simulink model "LKA_ensemble_RL_training"  (R2022a)
settings: Solver=FixedStepAuto  StartTime=0.0  StopTime=T  FixedStep=Ts  RelTol=1e-3
undefined symbols (not defined in the file): actionTable, actionUB, Cf, Cr, DiscIntNeverNeededParam, e1_initial, e2_initial, isEnsembleTerminate, isPred, isTerminate, Iz, lat_terminate_error, lf, lr, m, max_late_dev, max_rel_yaw_ang, md, rewardToIndex, rewardUB1, rewardUB2, rewardWeights, stateTable, tranTable, Ts, u_max, u_min, Vx
libraries: rllib x10, simulink x2
settings Model: Creator=The MathWorks, Inc.  LastModifiedBy=jiayangsong
settings SolverCC: AlgebraicLoopSolver=TrustRegion
settings DataIOCC: ReturnWorkspaceOutputs=off
settings DebuggingCC: UnconnectedInputMsg=warning  UnconnectedOutputMsg=warning  UnconnectedLineMsg=warning  SFMachineParentedDataDiag=warning  ArithmeticOperatorsInVariantConditions=warning
settings SFSimCC: SimUseLocalCustomCode=off  CustomCodeUndefinedFunction=UseInterfaceOnly
settings RTWCC: RTWUseLocalCustomCode=off  DLArmComputeVersion=19.05
settings CodeAppCC: StateflowObjectComments=on
settings SimscapeCC: SimscapeNormalizeSystem=off

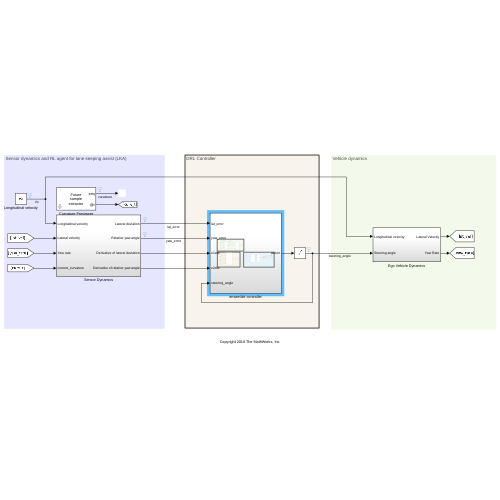
[thumbnail: Simulink's stored preview of the top-level diagram]
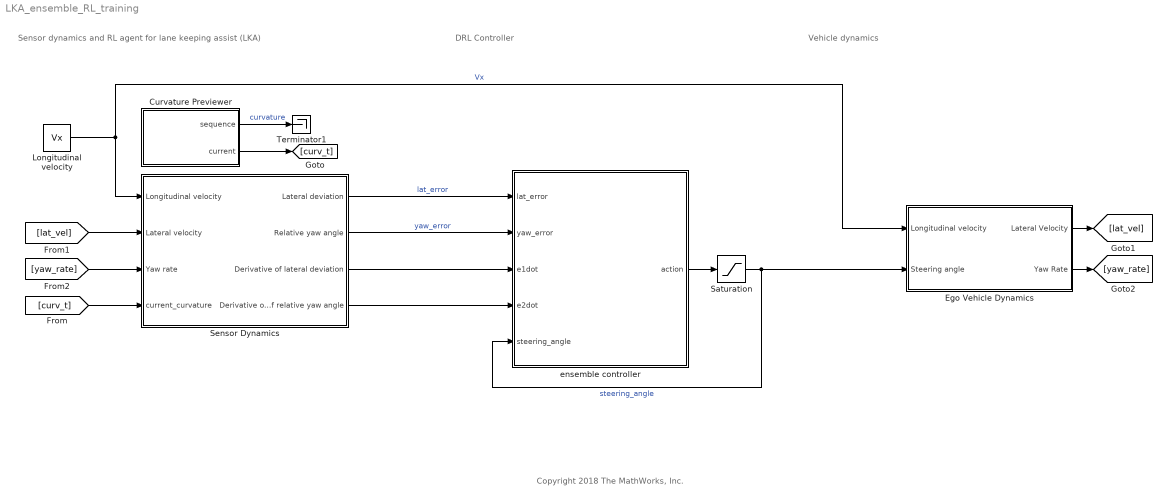
== system LKA_ensemble_RL_training ==
  note: DRL Controller
  note: Vehicle dynamics
  note: Sensor dynamics and RL agent for lane keeping assist (LKA)
  note: Copyright 2018 The MathWorks, Inc.
  Curvature Previewer : Subsystem  mask{signal=md, ts=Ts, steps=10}
      mask prompts: signal "Signal name"; ts "Sampling time"; steps "Number of previewing steps"
      mask init:
      | ts = evalin('base',get_param(gcbh,'ts'));
      | signal = evalin('base',get_param(gcbh,'signal'));
      | steps = evalin('base',get_param(gcbh,'steps'));
      | data = mpc_previewer_maskinit(signal,ts);
      mask Display:
      | fprintf('Future\nsample\nextractor');
      | port_label('output', 1, 'seq')
      | port_label('output', 2, '@t')
  Ego Vehicle Dynamics : Subsystem
  Longitudinal velocity : Constant  Value=Vx  SampleTime=Ts
  Saturation : Saturate  UpperLimit=u_max  LowerLimit=u_min
  Sensor Dynamics : Subsystem
  Terminator1 : Terminator
  ensemble controller : Subsystem
  wires:
  Ego Vehicle Dynamics/1(Lateral Velocity) -> [lat_vel]
  Longitudinal velocity/1 -> Ego Vehicle Dynamics/1(Longitudinal velocity), Sensor Dynamics/1(Longitudinal velocity)  "Vx"
  Curvature Previewer/2(current) -> [curv_t]
  [curv_t] -> Sensor Dynamics/4(current_curvature)
  Ego Vehicle Dynamics/2(Yaw Rate) -> [yaw_rate]
  [lat_vel] -> Sensor Dynamics/2(Lateral velocity)
  [yaw_rate] -> Sensor Dynamics/3(Yaw rate)
  Saturation/1 -> Ego Vehicle Dynamics/2(Steering angle), ensemble controller/5(steering_angle)  "steering_angle"
  Curvature Previewer/1(sequence) -> Terminator1/1  "curvature"
  Sensor Dynamics/1(Lateral deviation) -> ensemble controller/1(lat_error)  "lat_error"
  Sensor Dynamics/2(Relative yaw angle) -> ensemble controller/2(yaw_error)  "yaw_error"
  Sensor Dynamics/3(Derivative of lateral deviation) -> ensemble controller/3("e1dot ")
  Sensor Dynamics/4(Derivative of relative yaw angle) -> ensemble controller/4(e2dot)
  ensemble controller/1(action) -> Saturation/1

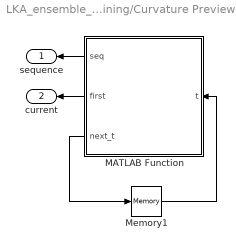
== system LKA_ensemble_RL_training/Curvature Previewer ==
  MATLAB Function : MATLAB Function  TreatAsAtomicUnit=on
  Memory1 : Memory  InheritSampleTime=on  LinearizeAsDelay=on
  sequence : Outport  VectorParamsAs1DForOutWhenUnconnected=off
  current : Outport  Port=2  VectorParamsAs1DForOutWhenUnconnected=off
  wires:
  MATLAB Function/1(seq) -> sequence/1
  MATLAB Function/2(first) -> current/1
  Memory1/1 -> MATLAB Function/1(t)
  MATLAB Function/3(next_t) -> Memory1/1

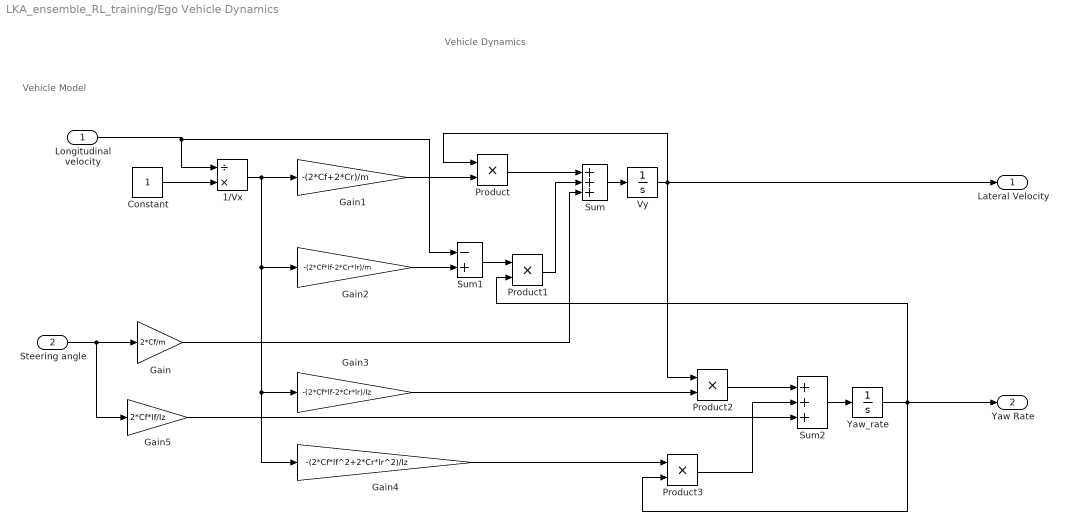
== system LKA_ensemble_RL_training/Ego Vehicle Dynamics ==
  note: Vehicle Model
  note: Vehicle Dynamics
  Longitudinal velocity : Inport
  Steering angle : Inport  Port=2
  1/Vx : Product  Inputs=/*
  Constant : Constant
  Gain : Gain  Gain=2*Cf/m
  Gain1 : Gain  Gain=-(2*Cf+2*Cr)/m
  Gain2 : Gain  Gain=-(2*Cf*lf-2*Cr*lr)/m
  Gain3 : Gain  Gain=-(2*Cf*lf-2*Cr*lr)/Iz
  Gain4 : Gain  Gain=-(2*Cf*lf^2+2*Cr*lr^2)/Iz
  Gain5 : Gain  Gain=2*Cf*lf/Iz
  Product{,1..3} (4 alike) : Product
  Sum : Sum  Inputs=+++
  Sum1 : Sum  Inputs=-+
  Sum2 : Sum  Inputs=+++
  Vy : Integrator
  "Yaw_rate " : Integrator
  Lateral Velocity : Outport  VectorParamsAs1DForOutWhenUnconnected=off
  Yaw Rate : Outport  Port=2  VectorParamsAs1DForOutWhenUnconnected=off
  wires:
  Sum2/1 -> "Yaw_rate "/1
  Gain2/1 -> Sum1/2
  Gain4/1 -> Product3/1
  Constant/1 -> 1/Vx/2
  Gain3/1 -> Product2/2
  1/Vx/1 -> Gain4/1, Gain3/1, Gain2/1, Gain1/1
  Product2/1 -> Sum2/1
  Product3/1 -> Sum2/2
  Gain5/1 -> Sum2/3
  Sum1/1 -> Product1/1
  "Yaw_rate "/1 -> Product3/2, Yaw Rate/1, Product1/2
  Gain/1 -> Sum/3
  Steering angle/1 -> Gain/1, Gain5/1
  Gain1/1 -> Product/2
  Product/1 -> Sum/1
  Vy/1 -> Product/1, Lateral Velocity/1, Product2/1
  Sum/1 -> Vy/1
  Longitudinal velocity/1 -> Sum1/1, 1/Vx/1
  Product1/1 -> Sum/2

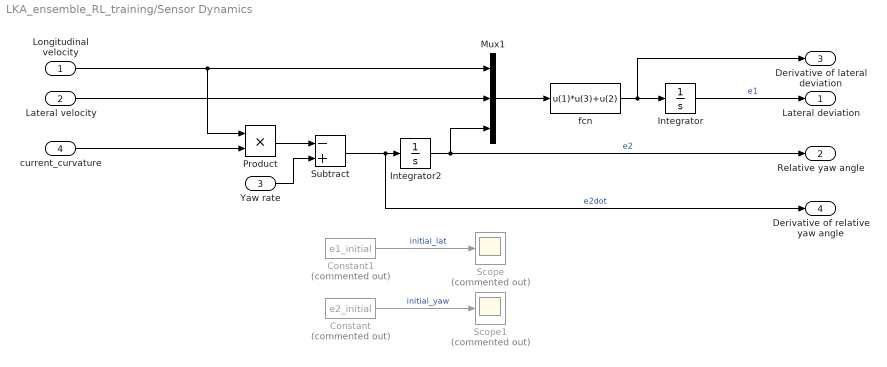
== system LKA_ensemble_RL_training/Sensor Dynamics ==
  Longitudinal velocity : Inport
  Lateral velocity : Inport  Port=2
  Yaw rate : Inport  Port=3
  current_curvature : Inport  Port=4
  Constant : Constant  Commented=on  Value=e2_initial
  Constant1 : Constant  Commented=on  Value=e1_initial
  Integrator : Integrator  InitialCondition=e1_initial
  Integrator2 : Integrator  InitialCondition=e2_initial
  Mux1 : Mux  Inputs=[1 1 1]
  Product : Product
  Scope : Scope  Commented=on
  Scope1 : Scope  Commented=on
  Subtract : Sum  Inputs=-+
  fcn : Fcn  Expr=u(1)*u(3)+u(2)
  Lateral deviation : Outport  VectorParamsAs1DForOutWhenUnconnected=off
  Relative yaw angle : Outport  Port=2  VectorParamsAs1DForOutWhenUnconnected=off
  Derivative of lateral deviation : Outport  Port=3  VectorParamsAs1DForOutWhenUnconnected=off
  Derivative of relative yaw angle : Outport  Port=4  VectorParamsAs1DForOutWhenUnconnected=off
  wires:
  Integrator2/1 -> Relative yaw angle/1, Mux1/3  "e2"
  Mux1/1 -> fcn/1
  fcn/1 -> Derivative of lateral deviation/1, Integrator/1
  Lateral velocity/1 -> Mux1/2
  Integrator/1 -> Lateral deviation/1  "e1"
  Product/1 -> Subtract/1
  Yaw rate/1 -> Subtract/2
  Subtract/1 -> Derivative of relative yaw angle/1, Integrator2/1  "e2dot"
  Longitudinal velocity/1 -> Mux1/1, Product/1
  current_curvature/1 -> Product/2
  Constant1/1 -> Scope/1  "initial_lat"
  Constant/1 -> Scope1/1  "initial_yaw"

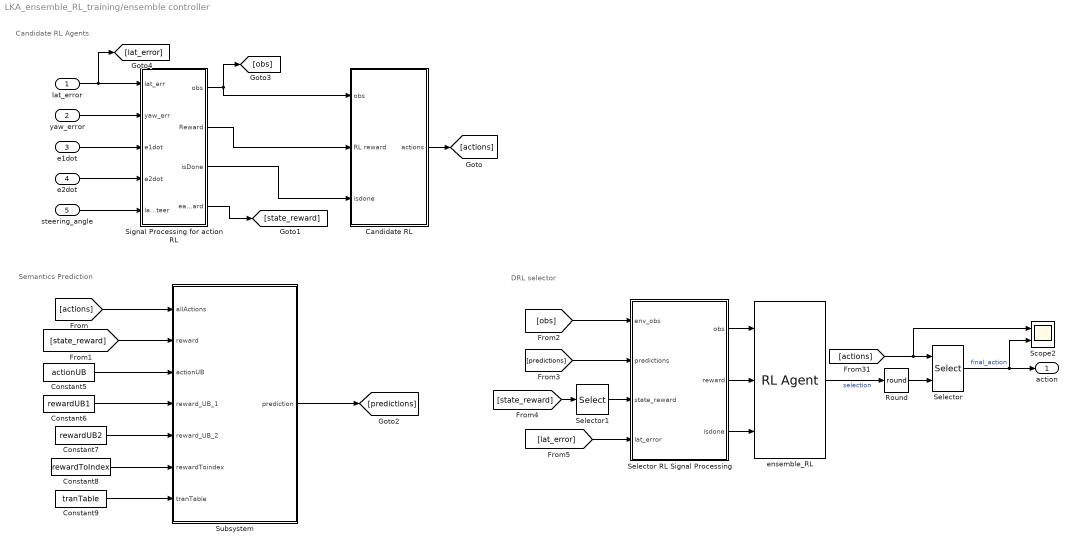
== system LKA_ensemble_RL_training/ensemble controller ==
  note: DRL selector
  note: Semantics Prediction
  note: Candidate RL Agents
  lat_error : Inport
  yaw_error : Inport  Port=2
  "e1dot " : Inport  Port=3
  e2dot : Inport  Port=4
  steering_angle : Inport  Port=5
  Candidate RL : Subsystem
  Constant5 : Constant  Value=actionUB
  Constant6 : Constant  Value=rewardUB1
  Constant7 : Constant  Value=rewardUB2
  Constant8 : Constant  Value=rewardToIndex
  Constant9 : Constant  Value=tranTable
  Round : Rounding  Operator=round
  Scope2 : Scope  NumInputPorts=2
  Selector : Selector  IndexOptions=Index vector (port)  Indices=[1 3]  OutputSizes=1
  Selector RL Signal Processing : Subsystem
  Selector1 : Selector  InputPortWidth=3  IndexOptions=Index vector (dialog)  Indices=[3]  OutputSizes=1
  "Signal Processing for action RL " : Subsystem
  Subsystem : Subsystem
  ensemble_RL : rllib/RL Agent  Agent=agentEnsemble  ExternalActionAsInput=off  ProvideLastAction=off  ProvideCumRwd=off  TreatAsDirectFeedthrough=on  UseStrictObservationDataTypes=off
  action : Outport
  wires:
  yaw_error/1 -> "Signal Processing for action RL "/2(yaw_err)
  e2dot/1 -> "Signal Processing for action RL "/4(e2dot)
  steering_angle/1 -> "Signal Processing for action RL "/5(last_RL_steer)
  "e1dot "/1 -> "Signal Processing for action RL "/3("e1dot ")
  lat_error/1 -> [lat_error], "Signal Processing for action RL "/1(lat_err)
  "Signal Processing for action RL "/1(obs) -> Candidate RL/1(obs), [obs]
  "Signal Processing for action RL "/2(Reward) -> Candidate RL/2(RL reward)
  "Signal Processing for action RL "/3(isDone) -> Candidate RL/3(isdone)
  Candidate RL/1(actions) -> [actions]
  [actions] -> Subsystem/1(allActions)
  [state_reward] -> Subsystem/2(reward)
  Constant5/1 -> Subsystem/3(actionUB)
  Constant7/1 -> Subsystem/5(reward_UB_2)
  Constant6/1 -> Subsystem/4(reward_UB_1)
  Constant8/1 -> Subsystem/6(rewardToindex)
  Constant9/1 -> Subsystem/7(tranTable)
  ensemble_RL/1 -> Round/1  "selection"
  Round/1 -> Selector/2
  [actions] -> Scope2/1, Selector/1
  Selector/1 -> Scope2/2, action/1  "final_action"
  Selector RL Signal Processing/1(obs) -> ensemble_RL/1
  Selector RL Signal Processing/2(reward) -> ensemble_RL/2
  Selector RL Signal Processing/3(isdone) -> ensemble_RL/3
  [obs] -> Selector RL Signal Processing/1(env_obs)
  [predictions] -> Selector RL Signal Processing/2(predictions)
  [lat_error] -> Selector RL Signal Processing/4(lat_error)
  Subsystem/1(prediction) -> [predictions]
  "Signal Processing for action RL "/4(each_reward) -> [state_reward]
  [state_reward] -> Selector1/1
  Selector1/1 -> Selector RL Signal Processing/3(state_reward)

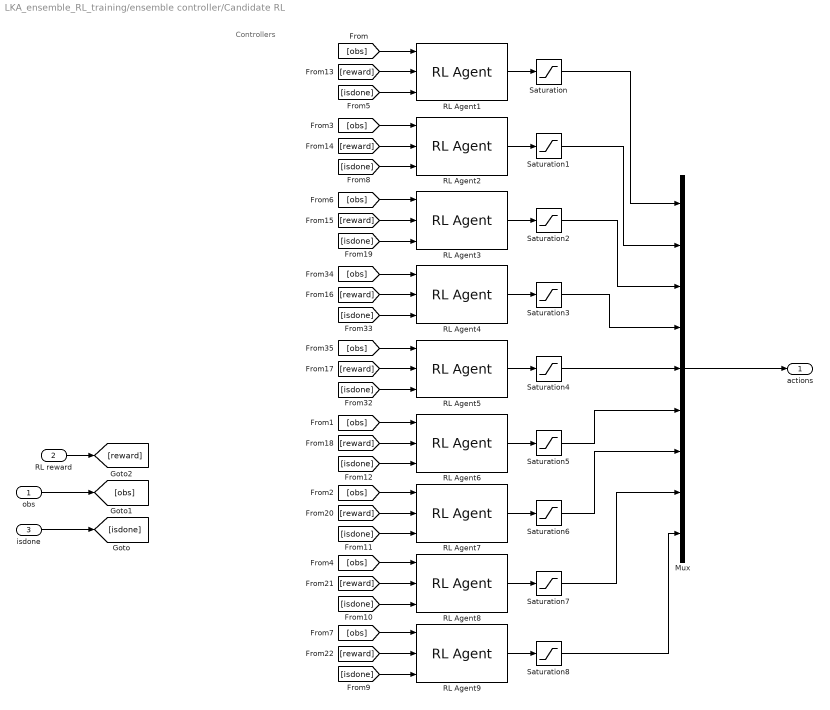
== system LKA_ensemble_RL_training/ensemble controller/Candidate RL ==
  note: Controllers
  obs : Inport
  RL reward : Inport  Port=2
  isdone : Inport  Port=3
  Mux : Mux  Inputs=9
  RL Agent1 : rllib/RL Agent  Agent=agent1  ExternalActionAsInput=off  ProvideLastAction=off  ProvideCumRwd=off  TreatAsDirectFeedthrough=on  UseStrictObservationDataTypes=off
  RL Agent2 : rllib/RL Agent  Agent=agent2  ExternalActionAsInput=off  ProvideLastAction=off  ProvideCumRwd=off  TreatAsDirectFeedthrough=on  UseStrictObservationDataTypes=off
  RL Agent3 : rllib/RL Agent  Agent=agent3  ExternalActionAsInput=off  ProvideLastAction=off  ProvideCumRwd=off  TreatAsDirectFeedthrough=on  UseStrictObservationDataTypes=off
  RL Agent4 : rllib/RL Agent  Agent=agent3  ExternalActionAsInput=off  ProvideLastAction=off  ProvideCumRwd=off  TreatAsDirectFeedthrough=on  UseStrictObservationDataTypes=off
  RL Agent5 : rllib/RL Agent  Agent=agent3  ExternalActionAsInput=off  ProvideLastAction=off  ProvideCumRwd=off  TreatAsDirectFeedthrough=on  UseStrictObservationDataTypes=off
  RL Agent6 : rllib/RL Agent  Agent=agent6  ExternalActionAsInput=off  ProvideLastAction=off  ProvideCumRwd=off  TreatAsDirectFeedthrough=on  UseStrictObservationDataTypes=off
  RL Agent7 : rllib/RL Agent  Agent=agent7  ExternalActionAsInput=off  ProvideLastAction=off  ProvideCumRwd=off  TreatAsDirectFeedthrough=on  UseStrictObservationDataTypes=off
  RL Agent8 : rllib/RL Agent  Agent=agent8  ExternalActionAsInput=off  ProvideLastAction=off  ProvideCumRwd=off  TreatAsDirectFeedthrough=on  UseStrictObservationDataTypes=off
  RL Agent9 : rllib/RL Agent  Agent=agent9  ExternalActionAsInput=off  ProvideLastAction=off  ProvideCumRwd=off  TreatAsDirectFeedthrough=on  UseStrictObservationDataTypes=off
  Saturation{,1..8} (9 alike) : Saturate  UpperLimit=u_max  LowerLimit=u_min
  actions : Outport
  wires:
  [obs] -> RL Agent7/1
  [obs] -> RL Agent4/1
  [obs] -> RL Agent3/1
  Saturation3/1 -> Mux/4
  [obs] -> RL Agent1/1
  [isdone] -> RL Agent1/3
  [obs] -> RL Agent2/1
  [obs] -> RL Agent5/1
  RL Agent1/1 -> Saturation/1
  [isdone] -> RL Agent8/3
  [isdone] -> RL Agent6/3
  Saturation/1 -> Mux/1
  RL Agent6/1 -> Saturation5/1
  Saturation4/1 -> Mux/5
  RL Agent3/1 -> Saturation2/1
  [isdone] -> RL Agent2/3
  [isdone] -> RL Agent7/3
  RL Agent8/1 -> Saturation7/1
  Saturation1/1 -> Mux/2
  [isdone] -> RL Agent5/3
  Mux/1 -> actions/1
  [obs] -> RL Agent6/1
  [isdone] -> RL Agent3/3
  RL Agent5/1 -> Saturation4/1
  RL Agent4/1 -> Saturation3/1
  RL Agent7/1 -> Saturation6/1
  RL Agent2/1 -> Saturation1/1
  [obs] -> RL Agent8/1
  Saturation2/1 -> Mux/3
  [isdone] -> RL Agent4/3
  RL Agent9/1 -> Saturation8/1
  [obs] -> RL Agent9/1
  [isdone] -> RL Agent9/3
  Saturation5/1 -> Mux/6
  Saturation6/1 -> Mux/7
  Saturation7/1 -> Mux/8
  Saturation8/1 -> Mux/9
  isdone/1 -> [isdone]
  obs/1 -> [obs]
  RL reward/1 -> [reward]
  [reward] -> RL Agent1/2
  [reward] -> RL Agent2/2
  [reward] -> RL Agent3/2
  [reward] -> RL Agent4/2
  [reward] -> RL Agent5/2
  [reward] -> RL Agent6/2
  [reward] -> RL Agent7/2
  [reward] -> RL Agent8/2
  [reward] -> RL Agent9/2

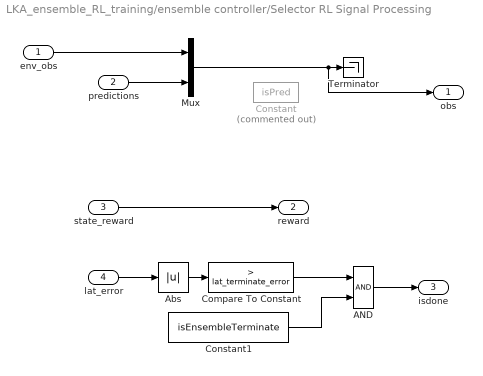
== system LKA_ensemble_RL_training/ensemble controller/Selector RL Signal Processing ==
  env_obs : Inport
  predictions : Inport  Port=2
  state_reward : Inport  Port=3
  lat_error : Inport  Port=4
  AND : Logic  IconShape=distinctive  AllPortsSameDT=off  OutDataTypeStr=boolean
  Abs : Abs  SaturateOnIntegerOverflow=off
  Compare To Constant : simulink/Logic and Bit Operations/Compare To Constant  relop=>  const=lat_terminate_error  OutDataTypeStr=boolean
  Constant : Constant  Commented=on  Value=isPred
  Constant1 : Constant  Value=isEnsembleTerminate
  Mux : Mux  Inputs=2
  Terminator : Terminator
  obs : Outport
  reward : Outport  Port=2
  isdone : Outport  Port=3
  wires:
  state_reward/1 -> reward/1
  Compare To Constant/1 -> AND/1
  Constant1/1 -> AND/2
  AND/1 -> isdone/1
  Abs/1 -> Compare To Constant/1
  lat_error/1 -> Abs/1
  predictions/1 -> Mux/2
  env_obs/1 -> Mux/1
  Mux/1 -> obs/1, Terminator/1

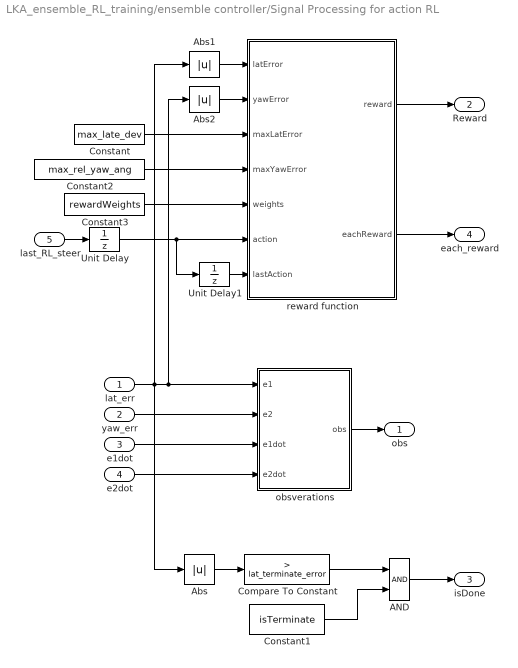
== system LKA_ensemble_RL_training/ensemble controller/Signal Processing for action RL  ==
  lat_err : Inport
  yaw_err : Inport  Port=2
  "e1dot " : Inport  Port=3
  e2dot : Inport  Port=4
  last_RL_steer : Inport  Port=5
  AND : Logic  IconShape=distinctive  AllPortsSameDT=off  OutDataTypeStr=boolean
  Abs : Abs  SaturateOnIntegerOverflow=off
  Abs1 : Abs  SaturateOnIntegerOverflow=off
  Abs2 : Abs  SaturateOnIntegerOverflow=off
  Compare To Constant : simulink/Logic and Bit Operations/Compare To Constant  relop=>  const=lat_terminate_error  OutDataTypeStr=boolean
  Constant : Constant  Value=max_late_dev
  Constant1 : Constant  Value=isTerminate
  Constant2 : Constant  Value=max_rel_yaw_ang
  Constant3 : Constant  Value=rewardWeights
  Unit Delay : UnitDelay  SampleTime=-1  HasFrameUpgradeWarning=on
  Unit Delay1 : UnitDelay  SampleTime=-1  HasFrameUpgradeWarning=on
  obsverations : Subsystem
  reward function : MATLAB Function  TreatAsAtomicUnit=on
  obs : Outport  VectorParamsAs1DForOutWhenUnconnected=off
  Reward : Outport  Port=2  VectorParamsAs1DForOutWhenUnconnected=off
  isDone : Outport  Port=3  VectorParamsAs1DForOutWhenUnconnected=off
  each_reward : Outport  Port=4
  wires:
  obsverations/1(obs) -> obs/1
  "e1dot "/1 -> obsverations/3(e1dot)
  e2dot/1 -> obsverations/4(e2dot)
  yaw_err/1 -> obsverations/2(e2)
  lat_err/1 -> obsverations/1(e1), Abs2/1, Abs1/1, Abs/1
  reward function/1(reward) -> Reward/1
  Constant/1 -> reward function/3(maxLatError)
  Abs1/1 -> reward function/1(latError)
  Abs2/1 -> reward function/2(yawError)
  last_RL_steer/1 -> Unit Delay/1
  Abs/1 -> Compare To Constant/1
  Compare To Constant/1 -> AND/1
  Constant1/1 -> AND/2
  AND/1 -> isDone/1
  Constant3/1 -> reward function/5(weights)
  Unit Delay1/1 -> reward function/7(lastAction)
  Constant2/1 -> reward function/4(maxYawError)
  Unit Delay/1 -> Unit Delay1/1, reward function/6(action)
  reward function/2(eachReward) -> each_reward/1

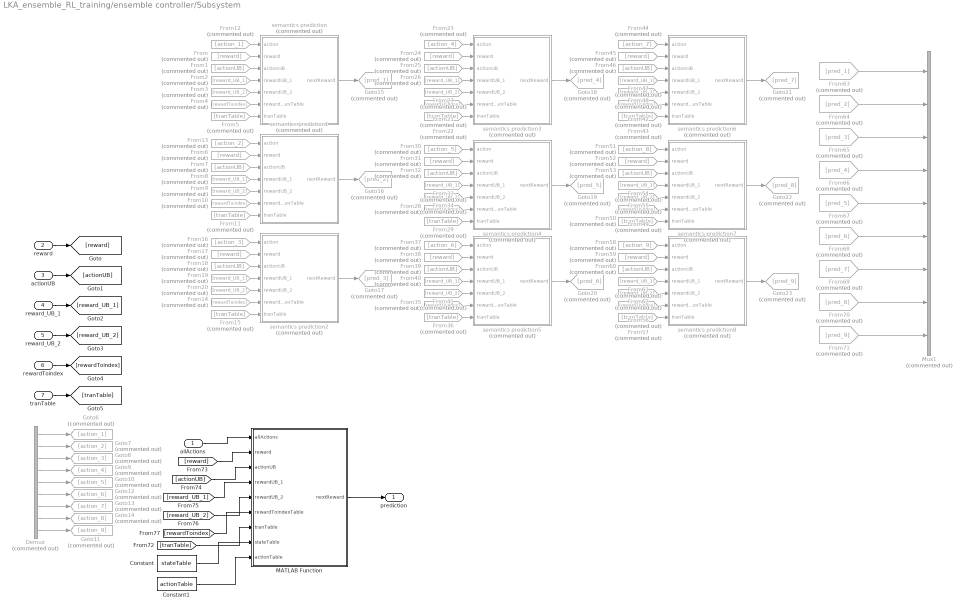
== system LKA_ensemble_RL_training/ensemble controller/Subsystem ==
  allActions : Inport
  reward : Inport  Port=2
  actionUB : Inport  Port=3
  reward_UB_1 : Inport  Port=4
  reward_UB_2 : Inport  Port=5
  rewardToindex : Inport  Port=6
  tranTable : Inport  Port=7
  Constant : Constant  Value=stateTable
  Constant1 : Constant  Value=actionTable
  Demux : Demux  Commented=on  Outputs=9
  From{,6,17,24,31,38,45,52,59} (9 alike) : From  Commented=on  GotoTag=reward
  From{1,7,18,25,32,39,46,53,60} (9 alike) : From  Commented=on  GotoTag=actionUB
  From{4,10,14,21,28,35,42,49,56} (9 alike) : From  Commented=on  GotoTag=rewardToindex
  From{5,11,15,22,29,36,43,50,57} (9 alike) : From  Commented=on  GotoTag=tranTable
  From12 : From  Commented=on  GotoTag=action_1
  From13 : From  Commented=on  GotoTag=action_2
  From16 : From  Commented=on  GotoTag=action_3
  From{2,8,19,26,33,40,47,54,61} (9 alike) : From  Commented=on  GotoTag=reward_UB_1
  From{3,9,20,27,34,41,48,55,62} (9 alike) : From  Commented=on  GotoTag=reward_UB_2
  From23 : From  Commented=on  GotoTag=action_4
  From30 : From  Commented=on  GotoTag=action_5
  From37 : From  Commented=on  GotoTag=action_6
  From44 : From  Commented=on  GotoTag=action_7
  From51 : From  Commented=on  GotoTag=action_8
  From58 : From  Commented=on  GotoTag=action_9
  From63 : From  Commented=on  GotoTag=pred_1
  From64 : From  Commented=on  GotoTag=pred_2
  From65 : From  Commented=on  GotoTag=pred_3
  From66 : From  Commented=on  GotoTag=pred_4
  From67 : From  Commented=on  GotoTag=pred_5
  From68 : From  Commented=on  GotoTag=pred_6
  From69 : From  Commented=on  GotoTag=pred_7
  From70 : From  Commented=on  GotoTag=pred_8
  From71 : From  Commented=on  GotoTag=pred_9
  Goto10 : Goto  Commented=on  GotoTag=action_5
  Goto11 : Goto  Commented=on  GotoTag=action_9
  Goto12 : Goto  Commented=on  GotoTag=action_6
  Goto13 : Goto  Commented=on  GotoTag=action_7
  Goto14 : Goto  Commented=on  GotoTag=action_8
  Goto15 : Goto  Commented=on  GotoTag=pred_1
  Goto16 : Goto  Commented=on  GotoTag=pred_2
  Goto17 : Goto  Commented=on  GotoTag=pred_3
  Goto18 : Goto  Commented=on  GotoTag=pred_4
  Goto19 : Goto  Commented=on  GotoTag=pred_5
  Goto20 : Goto  Commented=on  GotoTag=pred_6
  Goto21 : Goto  Commented=on  GotoTag=pred_7
  Goto22 : Goto  Commented=on  GotoTag=pred_8
  Goto23 : Goto  Commented=on  GotoTag=pred_9
  Goto6 : Goto  Commented=on  GotoTag=action_1
  Goto7 : Goto  Commented=on  GotoTag=action_2
  Goto8 : Goto  Commented=on  GotoTag=action_3
  Goto9 : Goto  Commented=on  GotoTag=action_4
  MATLAB Function : MATLAB Function  TreatAsAtomicUnit=on
  Mux1 : Mux  Commented=on  Inputs=9
  semantics prediction : MATLAB Function  Commented=on  TreatAsAtomicUnit=on
  semantics prediction1 : MATLAB Function  Commented=on  TreatAsAtomicUnit=on
  semantics prediction2 : MATLAB Function  Commented=on  TreatAsAtomicUnit=on
  semantics prediction3 : MATLAB Function  Commented=on  TreatAsAtomicUnit=on
  semantics prediction4 : MATLAB Function  Commented=on  TreatAsAtomicUnit=on
  semantics prediction5 : MATLAB Function  Commented=on  TreatAsAtomicUnit=on
  semantics prediction6 : MATLAB Function  Commented=on  TreatAsAtomicUnit=on
  semantics prediction7 : MATLAB Function  Commented=on  TreatAsAtomicUnit=on
  semantics prediction8 : MATLAB Function  Commented=on  TreatAsAtomicUnit=on
  prediction : Outport
  wires:
  reward/1 -> [reward]
  From/1 -> semantics prediction/2(reward)
  From63/1 -> Mux1/1
  From64/1 -> Mux1/2
  From65/1 -> Mux1/3
  From66/1 -> Mux1/4
  From67/1 -> Mux1/5
  From68/1 -> Mux1/6
  From69/1 -> Mux1/7
  From70/1 -> Mux1/8
  From71/1 -> Mux1/9
  actionUB/1 -> [actionUB]
  reward_UB_1/1 -> [reward_UB_1]
  reward_UB_2/1 -> [reward_UB_2]
  rewardToindex/1 -> [rewardToindex]
  tranTable/1 -> [tranTable]
  From1/1 -> semantics prediction/3(actionUB)
  From2/1 -> semantics prediction/4(rewardUB_1)
  From3/1 -> semantics prediction/5(rewardUB_2)
  From4/1 -> semantics prediction/6(rewardToIndexTable)
  From5/1 -> semantics prediction/7(tranTable)
  From9/1 -> semantics prediction1/5(rewardUB_2)
  From11/1 -> semantics prediction1/7(tranTable)
  From6/1 -> semantics prediction1/2(reward)
  From7/1 -> semantics prediction1/3(actionUB)
  From10/1 -> semantics prediction1/6(rewardToIndexTable)
  From8/1 -> semantics prediction1/4(rewardUB_1)
  Demux/1 -> Goto6/1
  Demux/2 -> Goto7/1
  Demux/3 -> Goto8/1
  Demux/4 -> Goto9/1
  Demux/5 -> Goto10/1
  Demux/6 -> Goto12/1
  Demux/7 -> Goto13/1
  Demux/8 -> Goto14/1
  Demux/9 -> Goto11/1
  From12/1 -> semantics prediction/1(action)
  From13/1 -> semantics prediction1/1(action)
  From16/1 -> semantics prediction2/1(action)
  From18/1 -> semantics prediction2/3(actionUB)
  From19/1 -> semantics prediction2/4(rewardUB_1)
  From14/1 -> semantics prediction2/6(rewardToIndexTable)
  From15/1 -> semantics prediction2/7(tranTable)
  From17/1 -> semantics prediction2/2(reward)
  From20/1 -> semantics prediction2/5(rewardUB_2)
  From23/1 -> semantics prediction3/1(action)
  From25/1 -> semantics prediction3/3(actionUB)
  From26/1 -> semantics prediction3/4(rewardUB_1)
  From21/1 -> semantics prediction3/6(rewardToIndexTable)
  From22/1 -> semantics prediction3/7(tranTable)
  From24/1 -> semantics prediction3/2(reward)
  From27/1 -> semantics prediction3/5(rewardUB_2)
  From30/1 -> semantics prediction4/1(action)
  From32/1 -> semantics prediction4/3(actionUB)
  From33/1 -> semantics prediction4/4(rewardUB_1)
  From28/1 -> semantics prediction4/6(rewardToIndexTable)
  From29/1 -> semantics prediction4/7(tranTable)
  From31/1 -> semantics prediction4/2(reward)
  From34/1 -> semantics prediction4/5(rewardUB_2)
  From37/1 -> semantics prediction5/1(action)
  From39/1 -> semantics prediction5/3(actionUB)
  From40/1 -> semantics prediction5/4(rewardUB_1)
  From35/1 -> semantics prediction5/6(rewardToIndexTable)
  From36/1 -> semantics prediction5/7(tranTable)
  From38/1 -> semantics prediction5/2(reward)
  From41/1 -> semantics prediction5/5(rewardUB_2)
  From50/1 -> semantics prediction7/7(tranTable)
  From53/1 -> semantics prediction7/3(actionUB)
  From52/1 -> semantics prediction7/2(reward)
  From47/1 -> semantics prediction6/4(rewardUB_1)
  From62/1 -> semantics prediction8/5(rewardUB_2)
  From56/1 -> semantics prediction8/6(rewardToIndexTable)
  From59/1 -> semantics prediction8/2(reward)
  From46/1 -> semantics prediction6/3(actionUB)
  From42/1 -> semantics prediction6/6(rewardToIndexTable)
  From57/1 -> semantics prediction8/7(tranTable)
  From44/1 -> semantics prediction6/1(action)
  From45/1 -> semantics prediction6/2(reward)
  From60/1 -> semantics prediction8/3(actionUB)
  From51/1 -> semantics prediction7/1(action)
  From48/1 -> semantics prediction6/5(rewardUB_2)
  From55/1 -> semantics prediction7/5(rewardUB_2)
  From61/1 -> semantics prediction8/4(rewardUB_1)
  From49/1 -> semantics prediction7/6(rewardToIndexTable)
  From43/1 -> semantics prediction6/7(tranTable)
  From54/1 -> semantics prediction7/4(rewardUB_1)
  From58/1 -> semantics prediction8/1(action)
  semantics prediction/1(nextReward) -> Goto15/1
  semantics prediction1/1(nextReward) -> Goto16/1
  semantics prediction2/1(nextReward) -> Goto17/1
  semantics prediction5/1(nextReward) -> Goto20/1
  semantics prediction4/1(nextReward) -> Goto19/1
  semantics prediction3/1(nextReward) -> Goto18/1
  semantics prediction8/1(nextReward) -> Goto23/1
  semantics prediction7/1(nextReward) -> Goto22/1
  semantics prediction6/1(nextReward) -> Goto21/1
  MATLAB Function/1(nextReward) -> prediction/1
  allActions/1 -> MATLAB Function/1(allActions)
  [reward] -> MATLAB Function/2(reward)
  [actionUB] -> MATLAB Function/3(actionUB)
  [reward_UB_1] -> MATLAB Function/4(rewardUB_1)
  [reward_UB_2] -> MATLAB Function/5(rewardUB_2)
  [rewardToindex] -> MATLAB Function/6(rewardToIndexTable)
  [tranTable] -> MATLAB Function/7(tranTable)
  Constant/1 -> MATLAB Function/8(stateTable)
  Constant1/1 -> MATLAB Function/9(actionTable)

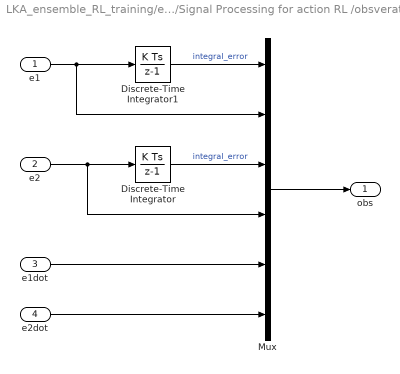
== system LKA_ensemble_RL_training/ensemble controller/Signal Processing for action RL /obsverations ==
  e1 : Inport
  e2 : Inport  Port=2
  e1dot : Inport  Port=3
  e2dot : Inport  Port=4
  Discrete-Time Integrator : DiscreteIntegrator  SampleTime=-1  ICPrevOutput=DiscIntNeverNeededParam  ICPrevScaledInput=DiscIntNeverNeededParam
  Discrete-Time Integrator1 : DiscreteIntegrator  SampleTime=-1  ICPrevOutput=DiscIntNeverNeededParam  ICPrevScaledInput=DiscIntNeverNeededParam
  Mux : Mux  Inputs=6
  obs : Outport  VectorParamsAs1DForOutWhenUnconnected=off
  wires:
  e1/1 -> Mux/2, Discrete-Time Integrator1/1
  Mux/1 -> obs/1
  Discrete-Time Integrator1/1 -> Mux/1  "integral_error"
  e2/1 -> Mux/4, Discrete-Time Integrator/1
  Discrete-Time Integrator/1 -> Mux/3  "integral_error"
  e1dot/1 -> Mux/5
  e2dot/1 -> Mux/6

== matlab function LKA_ensemble_RL_training/ensemble controller/Subsystem/semantics prediction4 ==
  data: nextReward output double; action input; reward input; actionUB input; rewardUB_1 input; rewardUB_2 input; rewardToIndexTable input; tranTable input
function nextReward  = fcn(action, reward,actionUB,rewardUB_1,rewardUB_2,rewardToIndexTable,tranTable)

nextReward = 0;

abReward_1 = find(rewardUB_1 >= reward(1), 1, 'first');  % concrete state -> abstract state
abReward_2 = find(rewardUB_2 >= reward(2), 1, 'first');
abState = rewardToIndexTable(rewardToIndexTable(:,1)==abReward_1 & rewardToIndexTable(:,2)==abReward_2,3);
stateTable = tranTable(:,1);
actionTable = tranTable(:,2);

abAction = find(actionUB >= action, 1, 'first');      % concrete action -> abstract action

if length(stateTable==abState) == length(actionTable==abAction)
    temp = (stateTable==abState) + (actionTable==abAction);
    if sum(temp == 2) ~=0
        pred_reward = tranTable((stateTable==abState & actionTable==abAction),3:5);
        nextReward= pred_reward(3);
    end
end

== matlab function LKA_ensemble_RL_training/ensemble controller/Subsystem/semantics prediction5 ==
  data: nextReward output double; action input; reward input; actionUB input; rewardUB_1 input; rewardUB_2 input; rewardToIndexTable input; tranTable input
function nextReward  = fcn(action, reward,actionUB,rewardUB_1,rewardUB_2,rewardToIndexTable,tranTable)

nextReward = 0;

abReward_1 = find(rewardUB_1 >= reward(1), 1, 'first');  % concrete state -> abstract state
abReward_2 = find(rewardUB_2 >= reward(2), 1, 'first');
abState = rewardToIndexTable(rewardToIndexTable(:,1)==abReward_1 & rewardToIndexTable(:,2)==abReward_2,3);
stateTable = tranTable(:,1);
actionTable = tranTable(:,2);

abAction = find(actionUB >= action, 1, 'first');      % concrete action -> abstract action

if length(stateTable==abState) == length(actionTable==abAction)
    temp = (stateTable==abState) + (actionTable==abAction);
    if sum(temp == 2) ~=0
        pred_reward = tranTable((stateTable==abState & actionTable==abAction),3:5);
        nextReward= pred_reward(3);
    end
end

== matlab function LKA_ensemble_RL_training/ensemble controller/Subsystem/semantics prediction6 ==
  data: nextReward output double; action input; reward input; actionUB input; rewardUB_1 input; rewardUB_2 input; rewardToIndexTable input; tranTable input
function nextReward  = fcn(action, reward,actionUB,rewardUB_1,rewardUB_2,rewardToIndexTable,tranTable)

nextReward = 0;

abReward_1 = find(rewardUB_1 >= reward(1), 1, 'first');  % concrete state -> abstract state
abReward_2 = find(rewardUB_2 >= reward(2), 1, 'first');
abState = rewardToIndexTable(rewardToIndexTable(:,1)==abReward_1 & rewardToIndexTable(:,2)==abReward_2,3);
stateTable = tranTable(:,1);
actionTable = tranTable(:,2);

abAction = find(actionUB >= action, 1, 'first');      % concrete action -> abstract action

if length(stateTable==abState) == length(actionTable==abAction)
    temp = (stateTable==abState) + (actionTable==abAction);
    if sum(temp == 2) ~=0
        pred_reward = tranTable((stateTable==abState & actionTable==abAction),3:5);
        nextReward= pred_reward(3);
    end
end

== matlab function LKA_ensemble_RL_training/ensemble controller/Subsystem/semantics prediction7 ==
  data: nextReward output double; action input; reward input; actionUB input; rewardUB_1 input; rewardUB_2 input; rewardToIndexTable input; tranTable input
function nextReward  = fcn(action, reward,actionUB,rewardUB_1,rewardUB_2,rewardToIndexTable,tranTable)

nextReward = 0;

abReward_1 = find(rewardUB_1 >= reward(1), 1, 'first');  % concrete state -> abstract state
abReward_2 = find(rewardUB_2 >= reward(2), 1, 'first');
abState = rewardToIndexTable(rewardToIndexTable(:,1)==abReward_1 & rewardToIndexTable(:,2)==abReward_2,3);
stateTable = tranTable(:,1);
actionTable = tranTable(:,2);

abAction = find(actionUB >= action, 1, 'first');      % concrete action -> abstract action

if length(stateTable==abState) == length(actionTable==abAction)
    temp = (stateTable==abState) + (actionTable==abAction);
    if sum(temp == 2) ~=0
        pred_reward = tranTable((stateTable==abState & actionTable==abAction),3:5);
        nextReward= pred_reward(3);
    end
end

== matlab function LKA_ensemble_RL_training/ensemble controller/Subsystem/semantics prediction8 ==
  data: nextReward output double; action input; reward input; actionUB input; rewardUB_1 input; rewardUB_2 input; rewardToIndexTable input; tranTable input
function nextReward  = fcn(action, reward,actionUB,rewardUB_1,rewardUB_2,rewardToIndexTable,tranTable)

nextReward = 0;

abReward_1 = find(rewardUB_1 >= reward(1), 1, 'first');  % concrete state -> abstract state
abReward_2 = find(rewardUB_2 >= reward(2), 1, 'first');
abState = rewardToIndexTable(rewardToIndexTable(:,1)==abReward_1 & rewardToIndexTable(:,2)==abReward_2,3);
stateTable = tranTable(:,1);
actionTable = tranTable(:,2);

abAction = find(actionUB >= action, 1, 'first');      % concrete action -> abstract action

if length(stateTable==abState) == length(actionTable==abAction)
    temp = (stateTable==abState) + (actionTable==abAction);
    if sum(temp == 2) ~=0
        pred_reward = tranTable((stateTable==abState & actionTable==abAction),3:5);
        nextReward= pred_reward(3);
    end
end

== matlab function LKA_ensemble_RL_training/ensemble controller/Subsystem/MATLAB Function ==
  data: allActions input; nextReward output; reward input; actionUB input; rewardUB_1 input; rewardUB_2 input; rewardToIndexTable input; tranTable input; stateTable input; actionTable input
function nextReward  = fcn(allActions, reward, actionUB, rewardUB_1,rewardUB_2, rewardToIndexTable, tranTable, stateTable,actionTable)

numController = 9;

nextReward = ones(numController, 1);
abReward_1 = find(rewardUB_1 >= reward(1), 1, 'first');  % concrete state -> abstract state
abReward_2 = find(rewardUB_2 >= reward(2), 1, 'first');

if isempty(abReward_1) || isempty(abReward_2)      % if this is an unseen reward
    nextReward = zeros(numController,1);
else
    rewardIndex1 = rewardToIndexTable(:,1)==abReward_1;
    rewardIndex2 = rewardToIndexTable(:,2)==abReward_2;
    
    if isempty(rewardIndex1) || isempty(rewardIndex2)      % if this is an unseen abstract state
        nextReward = zeros(numController,1);
    else
        abState = rewardToIndexTable(rewardToIndexTable(:,1)==abReward_1 & rewardToIndexTable(:,2)==abReward_2, 3);
        
        if isempty(abState)
            nextReward = zeros(numController,1);
        else
            for i = 1:numController
            
                action = allActions(i);
                abAction = find(actionUB >= action, 1, 'first');      % concrete action -> abstract action
            
                stateIndex = stateTable==abState;
                actionindex = actionTable==abAction;
            
                if isempty(stateIndex) || isempty(actionindex)  % if this is an unseen abstract state-action pair
                    abTranReward = 0;
                else
                    temp = stateIndex + actionindex;
                    if ismember(2,temp)
                        abTranReward = tranTable((stateIndex & actionindex),5);
                    else
                        abTranReward = 0;
                    end
                end
                nextReward(i,1) = abTranReward;
            end
        end
    end
end

== matlab function LKA_ensemble_RL_training/ensemble controller/Signal Processing for action RL /reward function ==
  data: latError input; reward output; yawError input; maxLatError input; maxYawError input; weights input; action input; lastAction input; eachReward output
function [reward,eachReward] = fcn(latError, yawError, maxLatError, maxYawError, weights, action, lastAction)


if latError <= maxLatError
    latReward = tanh(3*abs(maxLatError-latError));
else
    latReward = -tanh(3*abs(maxLatError-latError));
end


if yawError <= maxYawError
    yawReward = tanh(8*abs(maxYawError-yawError));
else
    yawReward = -tanh(9*abs(maxYawError-yawError));
end

stepReward = 0.05;
stableReward = -(action-lastAction)^2;

reward = weights(1)*latReward + weights(2)*yawReward + weights(3)*stableReward + stepReward;
eachReward = [latReward,yawReward,reward]';

== matlab function LKA_ensemble_RL_training/Curvature Previewer/MATLAB Function ==
  settings: updateMethod=DISCRETE  sampleTime=ts
  data: data parameter; seq output; steps parameter; t input; first output; next_t output
function [seq,first,next_t] = fcn(data,steps,t)
%#codegen
[seq,first,next_t] = mpcblock_preview('md',data,steps,t);

== matlab function LKA_ensemble_RL_training/ensemble controller/Subsystem/semantics prediction1 ==
  data: nextReward output double; action input; reward input; actionUB input; rewardUB_1 input; rewardUB_2 input; rewardToIndexTable input; tranTable input
function nextReward  = fcn(action, reward,actionUB,rewardUB_1,rewardUB_2,rewardToIndexTable,tranTable)

nextReward = 0;

abReward_1 = find(rewardUB_1 >= reward(1), 1, 'first');  % concrete state -> abstract state
abReward_2 = find(rewardUB_2 >= reward(2), 1, 'first');
abState = rewardToIndexTable(rewardToIndexTable(:,1)==abReward_1 & rewardToIndexTable(:,2)==abReward_2,3);
stateTable = tranTable(:,1);
actionTable = tranTable(:,2);

abAction = find(actionUB >= action, 1, 'first');      % concrete action -> abstract action

if length(stateTable==abState) == length(actionTable==abAction)
    temp = (stateTable==abState) + (actionTable==abAction);
    if sum(temp == 2) ~=0
        pred_reward = tranTable((stateTable==abState & actionTable==abAction),3:5);
        nextReward= pred_reward(3);
    end
end

== matlab function LKA_ensemble_RL_training/ensemble controller/Subsystem/semantics prediction ==
  data: nextReward output double; action input; reward input; actionUB input; rewardUB_1 input; rewardUB_2 input; rewardToIndexTable input; tranTable input
function nextReward  = fcn(action, reward,actionUB,rewardUB_1,rewardUB_2,rewardToIndexTable,tranTable)

nextReward = 0;

abReward_1 = find(rewardUB_1 >= reward(1), 1, 'first');  % concrete state -> abstract state
abReward_2 = find(rewardUB_2 >= reward(2), 1, 'first');
abState = rewardToIndexTable(rewardToIndexTable(:,1)==abReward_1 & rewardToIndexTable(:,2)==abReward_2,3);
stateTable = tranTable(:,1);
actionTable = tranTable(:,2);

abAction = find(actionUB >= action, 1, 'first');      % concrete action -> abstract action

if length(stateTable==abState) == length(actionTable==abAction)
    temp = (stateTable==abState) + (actionTable==abAction);
    if sum(temp == 2) ~=0
        pred_reward = tranTable((stateTable==abState & actionTable==abAction),3:5);
        nextReward= pred_reward(3);
    end
end

== matlab function LKA_ensemble_RL_training/ensemble controller/Subsystem/semantics prediction2 ==
  data: nextReward output double; action input; reward input; actionUB input; rewardUB_1 input; rewardUB_2 input; rewardToIndexTable input; tranTable input
function nextReward  = fcn(action, reward,actionUB,rewardUB_1,rewardUB_2,rewardToIndexTable,tranTable)

nextReward = 0;

abReward_1 = find(rewardUB_1 >= reward(1), 1, 'first');  % concrete state -> abstract state
abReward_2 = find(rewardUB_2 >= reward(2), 1, 'first');
abState = rewardToIndexTable(rewardToIndexTable(:,1)==abReward_1 & rewardToIndexTable(:,2)==abReward_2,3);
stateTable = tranTable(:,1);
actionTable = tranTable(:,2);

abAction = find(actionUB >= action, 1, 'first');      % concrete action -> abstract action

if length(stateTable==abState) == length(actionTable==abAction)
    temp = (stateTable==abState) + (actionTable==abAction);
    if sum(temp == 2) ~=0
        pred_reward = tranTable((stateTable==abState & actionTable==abAction),3:5);
        nextReward= pred_reward(3);
    end
end

== matlab function LKA_ensemble_RL_training/ensemble controller/Subsystem/semantics prediction3 ==
  data: nextReward output double; action input; reward input; actionUB input; rewardUB_1 input; rewardUB_2 input; rewardToIndexTable input; tranTable input
function nextReward  = fcn(action, reward,actionUB,rewardUB_1,rewardUB_2,rewardToIndexTable,tranTable)

nextReward = 0;

abReward_1 = find(rewardUB_1 >= reward(1), 1, 'first');  % concrete state -> abstract state
abReward_2 = find(rewardUB_2 >= reward(2), 1, 'first');
abState = rewardToIndexTable(rewardToIndexTable(:,1)==abReward_1 & rewardToIndexTable(:,2)==abReward_2,3);
stateTable = tranTable(:,1);
actionTable = tranTable(:,2);

abAction = find(actionUB >= action, 1, 'first');      % concrete action -> abstract action

if length(stateTable==abState) == length(actionTable==abAction)
    temp = (stateTable==abState) + (actionTable==abAction);
    if sum(temp == 2) ~=0
        pred_reward = tranTable((stateTable==abState & actionTable==abAction),3:5);
        nextReward= pred_reward(3);
    end
end
